simulink model "Bands8"  (R2018a)
settings: Solver=VariableStepAuto  StartTime=0.0  StopTime=0.007  RelTol=1e-3
undefined symbols (not defined in the file): fdesignblkfcn, G1, G2, G3, G4, G5, G6, G7, G8, gcbh, get, T
libraries: dspsrcs4 x1, dspxfrm3 x1, dspobslib x1
(part 3 of 3)

== system Bands8/Filter Bank /Filter 8/Bandpass Filter ==
  In : Inport
  Generated Filter Block : DiscreteFir  Tag=BlockMethodSubSystem  Coefficients=[-1.7502035522756131e-07 9.9986691463764788e-07 -3.21554516126294379e-06 7.19323112890193281e-06 -1.16443614212155322e-05 1.23553384460349571e-05 -2.51902715541787044e-06 -2.37164896632478877e-05 6.45553417156678684e-05 -0.000104068427219705745 0.000112168029091840306 -5.665940135771244e-05 -7.33144370864000425e-05 0.000243413376628060575 -0.000368678773356274849 0.000342545566025009558 -9.87037306211245612e-05 -0.000321927884808595054 0.000745156001002681193 -0.000916668987219297561 0.000632717632906146308 0.000109298912968679697 -0.00103481173517456842 0.0016685256852649558 -0.00156404835207463047 0.000584392012214246092 0.000933246114513488416 -0.0022643650127838681 0.00264149810648206789 -0.00169635403726306109 -0.000256378785813812543 0.00229741512716119577 -0.00335231837033949254 0.00278801101205320562 -0.000810183576006908422 -0.00159932335904584616 0.00320340776772162772 -0.00320050554302097646 0.00167313680064993696 0.00048396562528824614 -0.00211382962331074049 0.00247899333497248776 -0.00164521098686899302 0.000337552359551674427 0.000606587807631292692 -0.000796416823346534275 0.000474623919402225982 -0.000225466778251784671 0.000447133271462432343 -0.0010002346318829904 0.00130661871380040795 -0.000827583334735608489 -0.00044601275650191024 0.00188182087101118893 -0.00258674957788857483 0.00202245336967563907 -0.000408779058347478498 -0.0013886436622446523 0.00241626328727427087 -0.0022387048025627309 0.00116382634717706332 5.41833821259220434e-05 -0.000785055598653485289 0.000924803746374755703 -0.000839684096552329329 0.000934364514030131422 -0.00122653058652220362 0.00129747998831238748 -0.000672271785705273739 -0.000682972867952768041 0.00217655596289144338 -0.00291482827000166898 0.00232222246833778834 -0.000591283194856047161 -0.00139476010649123975 0.00262792148726776267 -0.00261624717629277371 0.0016308214725590923 -0.000401203454678863774 -0.000468787213480973807 0.000888783198536770335 -0.00118124848820138533 0.00162019315535371299 -0.00204374340632502245 0.0019113610044830798 -0.00078994679841548458 -0.00113600290739511271 0.00299448085900362072 -0.00372442761382837766 0.00280306346367350861 -0.000648316782994715632 -0.00162961722674881621 0.00295441959528122168 -0.00294335051386890355 0.00201712716037024146 -0.000923221053594268024 0.000103911053753016065 0.00055599113079712176 -0.00141362387205469118 0.00250211395845983389 -0.0032645541128843822 0.00289034156537756534 -0.00102506914019256847 -0.00174048451874508534 0.00407046273765969066 -0.00470235558320902195 0.00329529984069003344 -0.000659204860701882419 -0.0018180569845859286 0.0031028081412882466 -0.00309091555901115081 0.00241793952175020383 -0.00173336857132175 0.00110393266979414437 -7.53277501826227469e-05 -0.00167502472012237731 0.00371106576452844656 -0.00487364603231231312 0.00406369745274120196 -0.00118773576397931437 -0.00253186263460874507 0.00522134148079110919 -0.00555682382200030009 0.00360644526073814094 -0.000675521597568819621 -0.00170008084324054908 0.00279632807529822799 -0.00296306872955555672 0.00296631976086691659 -0.00305847750457904867 0.00265050301186728733 -0.000920230999868547513 -0.00216481841927937835 0.0053632124941925376 -0.00677246001140235226 0.00517450118388913111 -0.00106909656024615162 -0.00348526581327119386 0.00618562551427444436 -0.00598272579970412707 0.00362352671291225458 -0.000859733009092652307 -0.000979359851488531986 0.00185533286035646262 -0.00264528144477129377 0.003930553592345498 -0.00510316036739498751 0.00468459831485118928 -0.0016808043459314013 -0.00317974883891172268 0.00749520403761613253 -0.00868192177741683967 0.00583380722412289807 -0.000475493370742426243 -0.00444709017488152756 0.00659455829637785838 -0.00570625814677154161 0.00339581023317554352 -0.00153370085705855979 0.000646503001189963154 0.000283965255346773737 -0.00247856660147082559 0.00572132276017348756 -0.00799672581147510379 0.00691499163425061784 -0.00184688978501902309 -0.0050602891051488184 0.0100182251978241637 ...(+7229 chars)]  InputProcessing=Columns as channels (frame based)
  Out : Outport
  wires:
  In/1 -> Generated Filter Block/1
  Generated Filter Block/1 -> Out/1
